simulink library "cpc5"  (R2016a)
settings: Solver=ode45  StartTime=0.0  StopTime=10.0  RelTol=1e-3
undefined symbols (not defined in the file): sMP
libraries: CPC5_SFUN_wrapper x1
settings Model: Creator=ploch37  LastModifiedBy=PLOCH37
settings DataIOCC: LimitDataPoints=on
settings DebuggingCC: AllowSymbolicDim=off

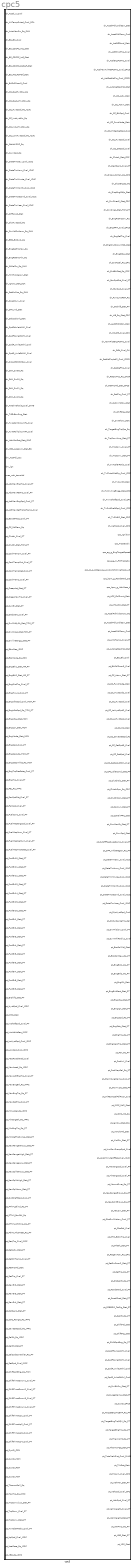
== system cpc5 ==
  cpc5 : Subsystem  mask{user_config=sMP.ctrl.cpc.user_config}
      mask prompts: user_config "Configuration String for S-Function"
      mask init:
      | cpc_mask_init;

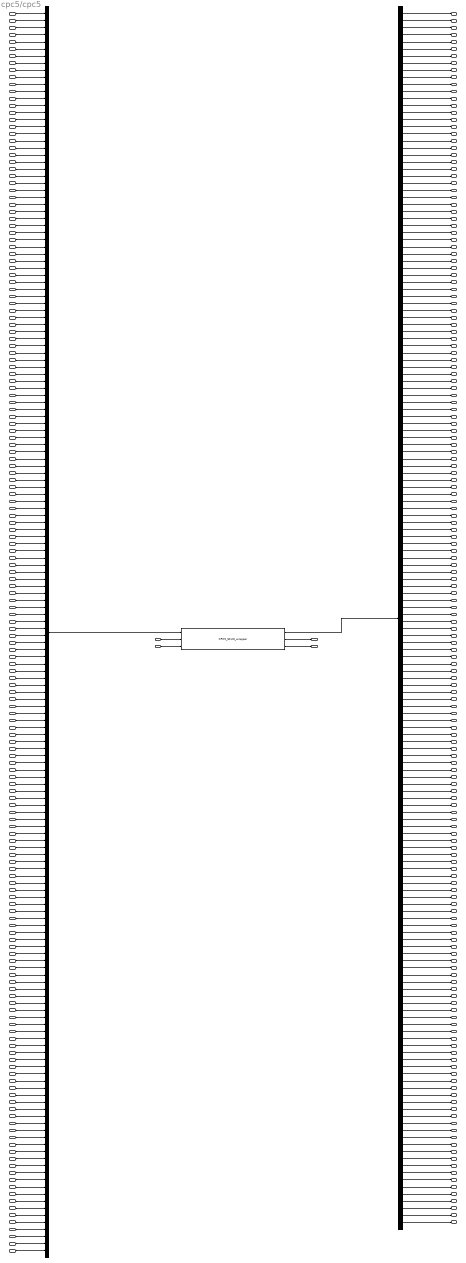
== system cpc5/cpc5 ==
  note: In- and Outports form a2lbus created with
      | cpc5_createPorts.m
      | from Spec folder in MKS.
      |
      | Ports sorted alphabetically with
      | slcSortPort.m
      | from tp/ead tools folder
  ch_Accel_X_Cval : Inport
  ch_AirTempOutsd_Cval_SCA : Inport  Port=2
  ch_AutoManSw_Rq_SAM : Inport  Port=3
  ch_BS_Brk_Cval : Inport  Port=4
  ch_BS_CSCPC_Acc_Stat : Inport  Port=5
  ch_BS_CSCPC_Intf_Stat : Inport  Port=6
  ch_BS_CSCPC_RqPerf_Stat : Inport  Port=7
  ch_BS_HB_RqPerf_Stat : Inport  Port=8
  ch_BrkPdlPosn3_Cval : Inport  Port=9
  ch_CC_DecHystSw_Rq : Inport  Port=10
  ch_CC_DecLoHystSw_Rq : Inport  Port=11
  ch_CC_HystSpd_Rq_ICUC : Inport  Port=12
  ch_CC_IncHystSw_Rq : Inport  Port=13
  ch_CC_IncLoHystSw_Rq : Inport  Port=14
  ch_CC_LowHystSpd_Rq_ICUC : Inport  Port=15
  ch_CstValIPPC_Rq : Inport  Port=16
  ch_CurvSpd_Rq : Inport  Port=17
  ch_DateTmDay_Cval_ICUC : Inport  Port=18
  ch_DateTmHour_Cval_ICUC : Inport  Port=19
  ch_DateTmMinute_Cval_ICUC : Inport  Port=20
  ch_DateTmMonth_Cval_ICUC : Inport  Port=21
  ch_DateTmSecond_Cval_ICUC : Inport  Port=22
  ch_DateTmYear_Cval_ICUC : Inport  Port=23
  ch_DiffLkIAC_Stat : Inport  Port=24
  ch_DipHystSpd_Rq : Inport  Port=25
  ch_DrvMdSwNorm_Rq_SAM : Inport  Port=26
  ch_EBS_BrkSw2_Rq : Inport  Port=27
  ch_EngRetTrqMax_Rq : Inport  Port=28
  ch_EngRetTrqMin_Rq : Inport  Port=29
  ch_GrSelSw_Rq_SAM : Inport  Port=30
  ch_HillHolderAvl_Stat : Inport  Port=31
  ch_IgnSw_Stat_SCA : Inport  Port=32
  ch_RetSwPos_Rq_SAM : Inport  Port=33
  ch_RoadCurv_Cval : Inport  Port=34
  ch_SFA_Ind_Stat : Inport  Port=35
  ch_SelSpdUnit_Stat : Inport  Port=36
  ch_SpdFtAxleLtWhl_Cval : Inport  Port=37
  ch_SpdFtAxleRtWhl_Cval : Inport  Port=38
  ch_SpdR_AxleLtWhl_Cval : Inport  Port=39
  ch_SpdR_AxleRtWhl_Cval : Inport  Port=40
  ch_SrcAdrBrkCtrlDev_Cval : Inport  Port=41
  ch_StW_Sw09_Rq : Inport  Port=42
  ch_StW_Sw10_Rq : Inport  Port=43
  ch_StW_Sw11_Rq : Inport  Port=44
  ch_StW_Sw13_Rq : Inport  Port=45
  ch_TotalVehDist_Cval_DIAG : Inport  Port=46
  ch_TrfGrBoxRng_Stat : Inport  Port=47
  ch_TyreRollCircumFA_Cval : Inport  Port=48
  ch_TyreRollCircumRA_Cval : Inport  Port=49
  ch_VehMtnDet_Stat_ICUC : Inport  Port=50
  ch_XBR_AccelLim_Stat_BS : Inport  Port=51
  drv_AccPdl_pos : Inport  Port=52
  drv_ign : Inport  Port=53
  mec_veh_transVel : Inport  Port=54
  pt_AbsMaxEngTrq_Cval_PT : Inport  Port=55
  pt_AbsMaxRetTrq_Cval_PT : Inport  Port=56
  pt_ActlMaxEngSpd_Cval_PT : Inport  Port=57
  pt_ActlMaxRetTrqNoTemp_Cval : Inport  Port=58
  pt_BoostPress_Cval_PT : Inport  Port=59
  pt_CC_MdDem_Rq : Inport  Port=60
  pt_Clutch_Cval_PT : Inport  Port=61
  pt_Clutch_Stat_TCM_PT : Inport  Port=62
  pt_CoolTempIn_Cval_PT : Inport  Port=63
  pt_CoolTempOut_Cval_PT : Inport  Port=64
  pt_CoolTempRet_Cval_PT : Inport  Port=65
  pt_CoolTemp_Cval_PT : Inport  Port=66
  pt_CreepAct_Stat_PT : Inport  Port=67
  pt_CreepMaxTrq_Cval_PT : Inport  Port=68
  pt_CurrGr_Stat_PT : Inport  Port=69
  pt_DeclSens_Cval_PT : Inport  Port=70
  pt_DrvDirByGr_Stat_TCM_PT : Inport  Port=71
  pt_DrvDirec_Stat_TCM_PT : Inport  Port=72
  pt_DrvlineEngg_Stat_PT : Inport  Port=73
  pt_EbmReq_IPPC : Inport  Port=74
  pt_EcoMode_Rq_PPC : Inport  Port=75
  pt_EngBrk1_Stat_MR_PT : Inport  Port=76
  pt_EngBrk2_Stat_MR_PT : Inport  Port=77
  pt_EngFrictTrq_Cval_PT : Inport  Port=78
  pt_EngHours_Cval_PT : Inport  Port=79
  pt_EngIdleSpd_Cval_MCM_PT : Inport  Port=80
  pt_EngIdleSpd_Rq_TCM_PT : Inport  Port=81
  pt_EngIdle_Stat_MCM : Inport  Port=82
  pt_EngIgn_Stat_MCM : Inport  Port=83
  pt_EngMode_Stat_MCM : Inport  Port=84
  pt_EngSpd_Cval_PT : Inport  Port=85
  pt_EngSpd_Rq_TCM_PT : Inport  Port=86
  pt_EngStSpInhbt_Rq_MCM : Inport  Port=87
  pt_EngTrqDecRate_Cval_PT : Inport  Port=88
  pt_EngTrq_Cval_PT : Inport  Port=89
  pt_FEL_Rq_IPPC : Inport  Port=90
  pt_FanSpdPct_Cval_PT : Inport  Port=91
  pt_FanSpd_Cval_PT : Inport  Port=92
  pt_FuelCons_Cval_PT : Inport  Port=93
  pt_FuelMapEngSpd_Cval_PT : Inport  Port=94
  pt_FuelMapNum_Cval_PT : Inport  Port=95
  pt_FuelMapSelNum_Cval_PT : Inport  Port=96
  pt_FuelMapTrqNoBst_Cval_PT : Inport  Port=97
  pt_FwdGr10_Stat_PT : Inport  Port=98
  pt_FwdGr11_Stat_PT : Inport  Port=99
  pt_FwdGr12_Stat_PT : Inport  Port=100
  pt_FwdGr13_Stat_PT : Inport  Port=101
  pt_FwdGr14_Stat_PT : Inport  Port=102
  pt_FwdGr15_Stat_PT : Inport  Port=103
  pt_FwdGr16_Stat_PT : Inport  Port=104
  pt_FwdGr1_Stat_PT : Inport  Port=105
  pt_FwdGr2_Stat_PT : Inport  Port=106
  pt_FwdGr3_Stat_PT : Inport  Port=107
  pt_FwdGr4_Stat_PT : Inport  Port=108
  pt_FwdGr5_Stat_PT : Inport  Port=109
  pt_FwdGr6_Stat_PT : Inport  Port=110
  pt_FwdGr7_Stat_PT : Inport  Port=111
  pt_FwdGr8_Stat_PT : Inport  Port=112
  pt_FwdGr9_Stat_PT : Inport  Port=113
  pt_GrShift_Stat_PT : Inport  Port=114
  pt_HystSpd_Cval_IPPC : Inport  Port=115
  pt_IPPC_Stat : Inport  Port=116
  pt_InShaftSpd_Cval_PT : Inport  Port=117
  pt_IntrUrbUcReq_IPPC : Inport  Port=118
  pt_LoHystSpd_Cval_IPPC : Inport  Port=119
  pt_LowSpd_Cval_IPPC : Inport  Port=120
  pt_MapRoadGrad_Cval : Inport  Port=121
  pt_MaxAccel_Rq_IPPC : Inport  Port=122
  pt_MaxActlEngTrq_Cval_PT : Inport  Port=123
  pt_MaxEngBrk_Rq_IPPC : Inport  Port=124
  pt_MaxEngTrq_Rq_PT : Inport  Port=125
  pt_MaxRetTrq_Cval_PT : Inport  Port=126
  pt_MinAccel_Rq_IPPC : Inport  Port=127
  pt_MinEngBrk_Rq_IPPC : Inport  Port=128
  pt_MinEngTrq_Rq_PT : Inport  Port=129
  pt_MinRetTrqPwrUp_Stat_PT : Inport  Port=130
  pt_NeuRangeGroup_Stat_PT : Inport  Port=131
  pt_NeuRangeHigh_Stat_PT : Inport  Port=132
  pt_NeuRangeLow_Stat_PT : Inport  Port=133
  pt_NeuSplitGroup_Stat_PT : Inport  Port=134
  pt_NeuSplitHigh_Stat_PT : Inport  Port=135
  pt_NeuSplitLow_Stat_PT : Inport  Port=136
  pt_OutShaftSpd_Cval_PT : Inport  Port=137
  pt_PThM_Blind_Rq_PT : Inport  Port=138
  pt_PThM_FanCtrl_Rq : Inport  Port=139
  pt_PThM_WtrPmp_Rq_PT : Inport  Port=140
  pt_PthM_ThstHeat_Rq_PT : Inport  Port=141
  pt_ReqTrq_Cval_IPPC : Inport  Port=142
  pt_RetActv_Stat_PT : Inport  Port=143
  pt_RetOilTemp_Cval_PT : Inport  Port=144
  pt_RetTrqMd_Stat : Inport  Port=145
  pt_RetTrq_Cval_PT : Inport  Port=146
  pt_RevGr2_Stat_PT : Inport  Port=147
  pt_RevGr3_Stat_PT : Inport  Port=148
  pt_RevGr4_Stat_PT : Inport  Port=149
  pt_RotSens_Stat_PT : Inport  Port=150
  pt_SOC_Range_Rq_IPPC : Inport  Port=151
  pt_SaveSetSpd_Rq_IPPC : Inport  Port=152
  pt_SelGr_Rq_IPPC : Inport  Port=153
  pt_SelGr_Stat_PT : Inport  Port=154
  pt_SelSpdController_Rq_PT : Inport  Port=155
  pt_SetSpd_Cval_IPPC : Inport  Port=156
  pt_ShiftSprtEng_Rq_TCM : Inport  Port=157
  pt_ShiftTimeDown1_Cval_PT : Inport  Port=158
  pt_ShiftTimeDown2_Cval_PT : Inport  Port=159
  pt_ShiftTimeDown3_Cval_PT : Inport  Port=160
  pt_ShiftTimeDown4_Cval_PT : Inport  Port=161
  pt_ShiftTimeUp1_Cval_PT : Inport  Port=162
  pt_ShiftTimeUp2_Cval_PT : Inport  Port=163
  pt_ShiftTimeUp3_Cval_PT : Inport  Port=164
  pt_ShiftTimeUp4_Cval_PT : Inport  Port=165
  pt_SysID_CCM : Inport  Port=166
  pt_SysID_MCM : Inport  Port=167
  pt_SysID_RCM : Inport  Port=168
  pt_SysID_TCM : Inport  Port=169
  pt_ThermoRoll_Rq : Inport  Port=170
  pt_TopTrq_Rq_IPPC : Inport  Port=171
  pt_TrqConvLkup_Stat_PT : Inport  Port=172
  pt_TrqConv_Cval_PT : Inport  Port=173
  pt_TrqConv_Stat_PT : Inport  Port=174
  pt_TxActlGrRatio_Cval_PT : Inport  Port=175
  pt_UpSpd_Cval_IPPC : Inport  Port=176
  pt_UseCase_Rq_IPPC : Inport  Port=177
  pt_XBR_Rq_IPPC : Inport  Port=178
  CPC5_SFUN_wrapper : CPC5_SFUN_wrapper/CPC5_SFUN_wrapper  SystemSampleTime=-1
  Inputs : BusCreator  Inputs=176
  Outputs : BusSelector  OutputSignals=out_ch_AccelPdlLoIdleSw_Stat,out_ch_AccelPdlPosn_Cval,out_ch_ActOffCond_Stat,out_ch_ActlEmotTrq_Cval,out_ch_ActlEngPctTrq_Cval,out_ch_ActlMaxAvlRetPctTrq_Cval_CPC3,out_ch_ActlRetPctTrq_Cval_CPC3,out_ch_AutoSetSpdMd_Stat,out_ch_CC_Actv_Stat,out_ch_CC_Actvn_Stat,out_ch_CC_BrkSpd_Cval,out_ch_CC_FuncMode_Stat,out_ch_CC_HiResSetSpd_Cval,out_ch_CC_HystSpd_Cval,out_ch_CC_SetSpd_Cval,out_ch_Clutch_Stat_CPC,out_ch_DeclSens_Cval_PT,out_ch_DispAutoMan_Rq_CPC,out_ch_DispEngSp_Rq,out_ch_DispEngStSp_Stat,out_ch_DrvDirec2_Stat_CPC,out_ch_DrvDirec_Stat_TCM_PT,out_ch_EngPctTrqDrv_Rq,out_ch_EngRPM_Cval_CPC3,out_ch_EngRefTrq_Cval,out_ch_EngShutDownMSS_Stat,out_ch_EngStSp_Stat,out_ch_ExtAccel_Rq_CPC,out_ch_ExtBrkStat_Rq_CPC,out_ch_FanSpdPct_Cval_PT,out_ch_FanSpd_Cval_PT,out_ch_FuncLmpRET_Rq,out_ch_GrShift_Stat_PT,out_ch_HB_Rq_Stat_CPC,out_ch_LastGrRlsRsn_Stat,out_ch_MC_E3_Cval_CPC,out_ch_NomFrictEngPctTrq_Cval,out_ch_PtRt_Cval_CH,out_ch_RetPctTrqActl2_Cval_CPC3,out_ch_RetRefTrq_Cval,out_ch_RetSwPos_Rq_STSR,out_ch_RetTrqMd_Stat_CPC3,out_ch_RetTrq_Cval_PT,out_ch_SLDrvMdSw_Stat,out_ch_ShiftPrg_Stat,out_ch_SrvBrkSw_Stat,out_ch_TargetEngTrqCpc_Rq,out_ch_TrqConvLkup_Stat_PT,out_ch_TrqConv_Cval_PT,out_ch_TrqConv_Stat_PT,out_ch_TxActlGrRatio_Cval,out_ch_TxClutchPctSlp_Cval_CPC,out_ch_TxCurrGr_Stat,out_ch_TxDrvlineEngg_Stat_CPC,out_ch_TxInShaftSpd_Cval_CPC,out_ch_TxOutShaftSpd_Cval_CPC,out_ch_TxShftIP_Stat_CPC,out_ch_VehSpd_Cval_CPC,out_pt_ACC_CtrlDmnt_Stat,out_pt_ATC_Ctrl_Stat_PT,out_pt_AccelPdlKickDnSw_Rq,out_pt_AccelPdlLoIdleSw_Stat,out_pt_AccelPdlPosn_Cval,out_pt_AmbTemp_Cval_PT,out_pt_AutoSetSpdMd_Stat,out_pt_BS_Brk_Cval,out_pt_BrkPdlPosn3_Cval,out_pt_CC_Actvn_Stat_PT,out_pt_CC_FuncMode_Stat,out_pt_CC_HystSpd2_Cval,out_pt_CC_HystSpd_Cval,out_pt_CC_LoHystSpd2_Cval,out_pt_CC_LoHystSpd_Cval,out_pt_CC_Md_Stat,out_pt_CC_SaveSetSpd_Rs,out_pt_CC_SetSpd3_Cval,out_pt_CC_SetSpd_Cval,out_pt_CC_SetSpd_Estm_Cval,out_pt_CPC_IdleCond_Stat_PT,out_pt_ClutchCls_Stat_PT,out_pt_ClutchOpn_Rq_CPC,out_pt_ClutchOpn_Stat_PT,out_pt_CoolLvl_Stat_PT,out_pt_CstValIPPC_Stat,out_pt_CurrManGr_Stat_PT,out_pt_CurvSpd_Stat,out_pt_CutoffFreqSurgDamp_Cval_PT,out_pt_DPF_InhbtRegen_Rq_PT,out_pt_DateTmDay_Cval_ICUC,out_pt_DateTmHour_Cval_ICUC,out_pt_DateTmMinute_Cval_ICUC,out_pt_DateTmMonth_Cval_ICUC,out_pt_DateTmSecond_Cval_ICUC,out_pt_DateTmYear_Cval_ICUC,out_pt_DipHystSpd_Cval,out_pt_DisturbanceTrq_Cal,out_pt_DrvFriction_Cval_PT,out_pt_DynWhlRadius_Cval,out_pt_EcoRollMd_Stat,out_pt_EcoRollNeu_Rq_PT,out_pt_EngBrk1_Rq_PT,out_pt_EngBrk2_Rq_PT,out_pt_EngCrk_Stat,out_pt_EngExtStart_Stat_PT,out_pt_EngIdle_Stat_PT,out_pt_EngIgn_Stat_PT,out_pt_EngSpd_Rq_PT,out_pt_EngStrtr_Stat_PT,out_pt_EngTrq_Rq_PT,out_pt_EngZeroTrq_Stat_PT,out_pt_Fan_Rq_PT,out_pt_FuelLvl_Cval,out_pt_FuelMapSel_Rq_PT,out_pt_GaimSurgDamp_Cval_PT,out_pt_GovType_Stat_PT,out_pt_HiResAccelPdlPosn_Cval,out_pt_IPPC_Md2_Stat,out_pt_IPPC_Md_Rq,out_pt_IgnSw_Stat_SCA,out_pt_IntrUrbMd_Stat,out_pt_KickDn_Stat_PT,out_pt_LimGovDroopSpd_Cval,out_pt_LocalMinuteOffset_Cval_ICUC,out_pt_MaxEngSpd_Cval_PT,out_pt_MinEngSpd_Cval_PT,out_pt_MomntOver_Rq_PT,out_pt_NeuRangeGroup_Rq_PT,out_pt_NeuSplitGroup_Rq_PT,out_pt_NeuSw_Stat_PT,out_pt_ObsDrvFriction_Cval_PT,out_pt_ObsSel_Cval,out_pt_PTO_EstmTrq_Cval,out_pt_PrkBrk_Stat_PT,out_pt_RegenActv_Rq_CPC,out_pt_RetSwPosn2_Stat_PT,out_pt_RetTrq_Rq_PT,out_pt_RlsSelGr_Rq_PT,out_pt_RoadGrad_Cval_PT,out_pt_RoadGrad_Stat_PT,out_pt_SPEEDO_ZeSig_Stat_PT,out_pt_SelGr_Rq_PT,out_pt_ShiftMd_Stat,out_pt_ShiftPrg_Stat,out_pt_ShiftSprtEng_Rq_PT,out_pt_SpdFtAxleLtWhl_Cval,out_pt_SpdFtAxleRtWhl_Cval,out_pt_SpdR_AxleLtWhl_Cval,out_pt_SpdR_AxleRtWhl_Cval,out_pt_SrvBrkSw_Stat_PT,out_pt_SurgeDamp_Stat_PT,out_pt_SysID_CPC3,out_pt_TargetEngTrqETP_Rq_PT,out_pt_TargetEngTrqRQV_Rq_PT,out_pt_TargetEngTrq_Rq_PT,out_pt_ThermoHt_Rq_PT,out_pt_ThermoMgt_Stat_PT,out_pt_TotalVehDist_Cval_DIAG,out_pt_TrlrDet_Stat,out_pt_TrqLim_Cval_CPC,out_pt_VehMtn_Stat_PT,out_pt_VehSpd_Cval_CPC,out_pt_VehSpd_Cval_PT,out_pt_VehWeight_Cval_PT,out_pt_VehWeight_Stat_PT,out_pt_WtrPmp_Rq_PT,out_pt_XBR_Stat_PT,out_pt_XSS_Stat,out_cpc_Ignition,out_cpc_TrqDecIdx,out_cpc_ag_g_EngTargetSpeed,out_cpc_ag_m_FiltTrqRatio,out_cpc_cc_p_CcSecure_LowSwitchOnVehSpd_u8
  ch_AccelPdlLoIdleSw_Stat : Outport
  ch_AccelPdlPosn_Cval : Outport  Port=2
  ch_ActOffCond_Stat : Outport  Port=3
  ch_ActlEmotTrq_Cval : Outport  Port=4
  ch_ActlEngPctTrq_Cval : Outport  Port=5
  ch_ActlMaxAvlRetPctTrq_Cval_CPC3 : Outport  Port=6
  ch_ActlRetPctTrq_Cval_CPC3 : Outport  Port=7
  ch_AutoSetSpdMd_Stat : Outport  Port=8
  ch_CC_Actv_Stat : Outport  Port=9
  ch_CC_Actvn_Stat : Outport  Port=10
  ch_CC_BrkSpd_Cval : Outport  Port=11
  ch_CC_FuncMode_Stat : Outport  Port=12
  ch_CC_HiResSetSpd_Cval : Outport  Port=13
  ch_CC_HystSpd_Cval : Outport  Port=14
  ch_CC_SetSpd_Cval : Outport  Port=15
  ch_Clutch_Stat_CPC : Outport  Port=16
  ch_DeclSens_Cval_PT : Outport  Port=17
  ch_DispAutoMan_Rq_CPC : Outport  Port=18
  ch_DispEngSp_Rq : Outport  Port=19
  ch_DispEngStSp_Stat : Outport  Port=20
  ch_DrvDirec2_Stat_CPC : Outport  Port=21
  ch_DrvDirec_Stat_TCM_PT : Outport  Port=22
  ch_EngPctTrqDrv_Rq : Outport  Port=23
  ch_EngRPM_Cval_CPC3 : Outport  Port=24
  ch_EngRefTrq_Cval : Outport  Port=25
  ch_EngShutDownMSS_Stat : Outport  Port=26
  ch_EngStSp_Stat : Outport  Port=27
  ch_ExtAccel_Rq_CPC : Outport  Port=28
  ch_ExtBrkStat_Rq_CPC : Outport  Port=29
  ch_FanSpdPct_Cval_PT : Outport  Port=30
  ch_FanSpd_Cval_PT : Outport  Port=31
  ch_FuncLmpRET_Rq : Outport  Port=32
  ch_GrShift_Stat_PT : Outport  Port=33
  ch_HB_Rq_Stat_CPC : Outport  Port=34
  ch_LastGrRlsRsn_Stat : Outport  Port=35
  ch_MC_E3_Cval_CPC : Outport  Port=36
  ch_NomFrictEngPctTrq_Cval : Outport  Port=37
  ch_PtRt_Cval_CH : Outport  Port=38
  ch_RetPctTrqActl2_Cval_CPC3 : Outport  Port=39
  ch_RetRefTrq_Cval : Outport  Port=40
  ch_RetSwPos_Rq_STSR : Outport  Port=41
  ch_RetTrqMd_Stat_CPC3 : Outport  Port=42
  ch_RetTrq_Cval_PT : Outport  Port=43
  ch_SLDrvMdSw_Stat : Outport  Port=44
  ch_ShiftPrg_Stat : Outport  Port=45
  ch_SrvBrkSw_Stat : Outport  Port=46
  ch_TargetEngTrqCpc_Rq : Outport  Port=47
  ch_TrqConvLkup_Stat_PT : Outport  Port=48
  ch_TrqConv_Cval_PT : Outport  Port=49
  ch_TrqConv_Stat_PT : Outport  Port=50
  ch_TxActlGrRatio_Cval : Outport  Port=51
  ch_TxClutchPctSlp_Cval_CPC : Outport  Port=52
  ch_TxCurrGr_Stat : Outport  Port=53
  ch_TxDrvlineEngg_Stat_CPC : Outport  Port=54
  ch_TxInShaftSpd_Cval_CPC : Outport  Port=55
  ch_TxOutShaftSpd_Cval_CPC : Outport  Port=56
  ch_TxShftIP_Stat_CPC : Outport  Port=57
  ch_VehSpd_Cval_CPC : Outport  Port=58
  cpc_Ignition : Outport  Port=59
  cpc_TrqDecIdx : Outport  Port=60
  cpc_ag_g_EngTargetSpeed : Outport  Port=61
  cpc_ag_m_FiltTrqRatio : Outport  Port=62
  cpc_cc_p_CcSecure_LowSwitchOnVehSpd_u8 : Outport  Port=63
  cpc_itpm_g_RoadGrad_pct : Outport  Port=64
  cpc_itpm_g_VehMass_t : Outport  Port=65
  pt_ACC_CtrlDmnt_Stat : Outport  Port=66
  pt_ATC_Ctrl_Stat_PT : Outport  Port=67
  pt_AccelPdlKickDnSw_Rq : Outport  Port=68
  pt_AccelPdlLoIdleSw_Stat : Outport  Port=69
  pt_AccelPdlPosn_Cval : Outport  Port=70
  pt_AmbTemp_Cval_PT : Outport  Port=71
  pt_AutoSetSpdMd_Stat : Outport  Port=72
  pt_BS_Brk_Cval : Outport  Port=73
  pt_BrkPdlPosn3_Cval : Outport  Port=74
  pt_CC_Actvn_Stat_PT : Outport  Port=75
  pt_CC_FuncMode_Stat : Outport  Port=76
  pt_CC_HystSpd2_Cval : Outport  Port=77
  pt_CC_HystSpd_Cval : Outport  Port=78
  pt_CC_LoHystSpd2_Cval : Outport  Port=79
  pt_CC_LoHystSpd_Cval : Outport  Port=80
  pt_CC_Md_Stat : Outport  Port=81
  pt_CC_SaveSetSpd_Rs : Outport  Port=82
  pt_CC_SetSpd3_Cval : Outport  Port=83
  pt_CC_SetSpd_Cval : Outport  Port=84
  pt_CC_SetSpd_Estm_Cval : Outport  Port=85
  pt_CPC_IdleCond_Stat_PT : Outport  Port=86
  pt_ClutchCls_Stat_PT : Outport  Port=87
  pt_ClutchOpn_Rq_CPC : Outport  Port=88
  pt_ClutchOpn_Stat_PT : Outport  Port=89
  pt_CoolLvl_Stat_PT : Outport  Port=90
  pt_CstValIPPC_Stat : Outport  Port=91
  pt_CurrManGr_Stat_PT : Outport  Port=92
  pt_CurvSpd_Stat : Outport  Port=93
  pt_CutoffFreqSurgDamp_Cval_PT : Outport  Port=94
  pt_DPF_InhbtRegen_Rq_PT : Outport  Port=95
  pt_DateTmDay_Cval_ICUC : Outport  Port=96
  pt_DateTmHour_Cval_ICUC : Outport  Port=97
  pt_DateTmMinute_Cval_ICUC : Outport  Port=98
  pt_DateTmMonth_Cval_ICUC : Outport  Port=99
  pt_DateTmSecond_Cval_ICUC : Outport  Port=100
  pt_DateTmYear_Cval_ICUC : Outport  Port=101
  pt_DipHystSpd_Cval : Outport  Port=102
  pt_DisturbanceTrq_Cal : Outport  Port=103
  pt_DrvFriction_Cval_PT : Outport  Port=104
  pt_DynWhlRadius_Cval : Outport  Port=105
  pt_EcoRollMd_Stat : Outport  Port=106
  pt_EcoRollNeu_Rq_PT : Outport  Port=107
  pt_EngBrk1_Rq_PT : Outport  Port=108
  pt_EngBrk2_Rq_PT : Outport  Port=109
  pt_EngCrk_Stat : Outport  Port=110
  pt_EngExtStart_Stat_PT : Outport  Port=111
  pt_EngIdle_Stat_PT : Outport  Port=112
  pt_EngIgn_Stat_PT : Outport  Port=113
  pt_EngSpd_Rq_PT : Outport  Port=114
  pt_EngStrtr_Stat_PT : Outport  Port=115
  pt_EngTrq_Rq_PT : Outport  Port=116
  pt_EngZeroTrq_Stat_PT : Outport  Port=117
  pt_Fan_Rq_PT : Outport  Port=118
  pt_FuelLvl_Cval : Outport  Port=119
  pt_FuelMapSel_Rq_PT : Outport  Port=120
  pt_GaimSurgDamp_Cval_PT : Outport  Port=121
  pt_GovType_Stat_PT : Outport  Port=122
  pt_HiResAccelPdlPosn_Cval : Outport  Port=123
  pt_IPPC_Md2_Stat : Outport  Port=124
  pt_IPPC_Md_Rq : Outport  Port=125
  pt_IgnSw_Stat_SCA : Outport  Port=126
  pt_IntrUrbMd_Stat : Outport  Port=127
  pt_KickDn_Stat_PT : Outport  Port=128
  pt_LimGovDroopSpd_Cval : Outport  Port=129
  pt_LocalMinuteOffset_Cval_ICUC : Outport  Port=130
  pt_MaxEngSpd_Cval_PT : Outport  Port=131
  pt_MinEngSpd_Cval_PT : Outport  Port=132
  pt_MomntOver_Rq_PT : Outport  Port=133
  pt_NeuRangeGroup_Rq_PT : Outport  Port=134
  pt_NeuSplitGroup_Rq_PT : Outport  Port=135
  pt_NeuSw_Stat_PT : Outport  Port=136
  pt_ObsDrvFriction_Cval_PT : Outport  Port=137
  pt_ObsSel_Cval : Outport  Port=138
  pt_PTO_EstmTrq_Cval : Outport  Port=139
  pt_PrkBrk_Stat_PT : Outport  Port=140
  pt_RegenActv_Rq_CPC : Outport  Port=141
  pt_RetSwPosn2_Stat_PT : Outport  Port=142
  pt_RetTrq_Rq_PT : Outport  Port=143
  pt_RlsSelGr_Rq_PT : Outport  Port=144
  pt_RoadGrad_Cval_PT : Outport  Port=145
  pt_RoadGrad_Stat_PT : Outport  Port=146
  pt_SPEEDO_ZeSig_Stat_PT : Outport  Port=147
  pt_SelGr_Rq_PT : Outport  Port=148
  pt_ShiftMd_Stat : Outport  Port=149
  pt_ShiftPrg_Stat : Outport  Port=150
  pt_ShiftSprtEng_Rq_PT : Outport  Port=151
  pt_SpdFtAxleLtWhl_Cval : Outport  Port=152
  pt_SpdFtAxleRtWhl_Cval : Outport  Port=153
  pt_SpdR_AxleLtWhl_Cval : Outport  Port=154
  pt_SpdR_AxleRtWhl_Cval : Outport  Port=155
  pt_SrvBrkSw_Stat_PT : Outport  Port=156
  pt_SurgeDamp_Stat_PT : Outport  Port=157
  pt_SysID_CPC3 : Outport  Port=158
  pt_TargetEngTrqETP_Rq_PT : Outport  Port=159
  pt_TargetEngTrqRQV_Rq_PT : Outport  Port=160
  pt_TargetEngTrq_Rq_PT : Outport  Port=161
  pt_ThermoHt_Rq_PT : Outport  Port=162
  pt_ThermoMgt_Stat_PT : Outport  Port=163
  pt_TotalVehDist_Cval_DIAG : Outport  Port=164
  pt_TrlrDet_Stat : Outport  Port=165
  pt_TrqLim_Cval_CPC : Outport  Port=166
  pt_VehMtn_Stat_PT : Outport  Port=167
  pt_VehSpd_Cval_CPC : Outport  Port=168
  pt_VehSpd_Cval_PT : Outport  Port=169
  pt_VehWeight_Cval_PT : Outport  Port=170
  pt_VehWeight_Stat_PT : Outport  Port=171
  pt_WtrPmp_Rq_PT : Outport  Port=172
  pt_XBR_Stat_PT : Outport  Port=173
  pt_XSS_Stat : Outport  Port=174
  wires:
  drv_AccPdl_pos/1 -> CPC5_SFUN_wrapper/2
  mec_veh_transVel/1 -> CPC5_SFUN_wrapper/3
  CPC5_SFUN_wrapper/2 -> cpc_itpm_g_RoadGrad_pct/1
  CPC5_SFUN_wrapper/3 -> cpc_itpm_g_VehMass_t/1
  ch_Accel_X_Cval/1 -> Inputs/1  "ch_Accel_X_Cval"
  ch_AirTempOutsd_Cval_SCA/1 -> Inputs/2  "ch_AirTempOutsd_Cval_SCA"
  ch_AutoManSw_Rq_SAM/1 -> Inputs/3  "ch_AutoManSw_Rq_SAM"
  ch_BS_Brk_Cval/1 -> Inputs/4  "ch_BS_Brk_Cval"
  ch_BS_CSCPC_Acc_Stat/1 -> Inputs/5  "ch_BS_CSCPC_Acc_Stat"
  ch_BS_CSCPC_Intf_Stat/1 -> Inputs/6  "ch_BS_CSCPC_Intf_Stat"
  ch_BS_CSCPC_RqPerf_Stat/1 -> Inputs/7  "ch_BS_CSCPC_RqPerf_Stat"
  ch_BS_HB_RqPerf_Stat/1 -> Inputs/8  "ch_BS_HB_RqPerf_Stat"
  ch_BrkPdlPosn3_Cval/1 -> Inputs/9  "ch_BrkPdlPosn3_Cval"
  ch_CC_DecHystSw_Rq/1 -> Inputs/10  "ch_CC_DecHystSw_Rq"
  ch_CC_DecLoHystSw_Rq/1 -> Inputs/11  "ch_CC_DecLoHystSw_Rq"
  ch_CC_HystSpd_Rq_ICUC/1 -> Inputs/12  "ch_CC_HystSpd_Rq_ICUC"
  ch_CC_IncHystSw_Rq/1 -> Inputs/13  "ch_CC_IncHystSw_Rq"
  ch_CC_IncLoHystSw_Rq/1 -> Inputs/14  "ch_CC_IncLoHystSw_Rq"
  ch_CC_LowHystSpd_Rq_ICUC/1 -> Inputs/15  "ch_CC_LowHystSpd_Rq_ICUC"
  ch_CstValIPPC_Rq/1 -> Inputs/16  "ch_CstValIPPC_Rq"
  ch_CurvSpd_Rq/1 -> Inputs/17  "ch_CurvSpd_Rq"
  ch_DateTmDay_Cval_ICUC/1 -> Inputs/18  "ch_DateTmDay_Cval_ICUC"
  ch_DateTmHour_Cval_ICUC/1 -> Inputs/19  "ch_DateTmHour_Cval_ICUC"
  ch_DateTmMinute_Cval_ICUC/1 -> Inputs/20  "ch_DateTmMinute_Cval_ICUC"
  ch_DateTmMonth_Cval_ICUC/1 -> Inputs/21  "ch_DateTmMonth_Cval_ICUC"
  ch_DateTmSecond_Cval_ICUC/1 -> Inputs/22  "ch_DateTmSecond_Cval_ICUC"
  ch_DateTmYear_Cval_ICUC/1 -> Inputs/23  "ch_DateTmYear_Cval_ICUC"
  ch_DiffLkIAC_Stat/1 -> Inputs/24  "ch_DiffLkIAC_Stat"
  ch_DipHystSpd_Rq/1 -> Inputs/25  "ch_DipHystSpd_Rq"
  ch_DrvMdSwNorm_Rq_SAM/1 -> Inputs/26  "ch_DrvMdSwNorm_Rq_SAM"
  ch_EBS_BrkSw2_Rq/1 -> Inputs/27  "ch_EBS_BrkSw2_Rq"
  ch_EngRetTrqMax_Rq/1 -> Inputs/28  "ch_EngRetTrqMax_Rq"
  ch_EngRetTrqMin_Rq/1 -> Inputs/29  "ch_EngRetTrqMin_Rq"
  ch_GrSelSw_Rq_SAM/1 -> Inputs/30  "ch_GrSelSw_Rq_SAM"
  ch_HillHolderAvl_Stat/1 -> Inputs/31  "ch_HillHolderAvl_Stat"
  ch_IgnSw_Stat_SCA/1 -> Inputs/32  "ch_IgnSw_Stat_SCA"
  ch_RetSwPos_Rq_SAM/1 -> Inputs/33  "ch_RetSwPos_Rq_SAM"
  ch_RoadCurv_Cval/1 -> Inputs/34  "ch_RoadCurv_Cval"
  ch_SFA_Ind_Stat/1 -> Inputs/35  "ch_SFA_Ind_Stat"
  ch_SelSpdUnit_Stat/1 -> Inputs/36  "ch_SelSpdUnit_Stat"
  ch_SpdFtAxleLtWhl_Cval/1 -> Inputs/37  "ch_SpdFtAxleLtWhl_Cval"
  ch_SpdFtAxleRtWhl_Cval/1 -> Inputs/38  "ch_SpdFtAxleRtWhl_Cval"
  ch_SpdR_AxleLtWhl_Cval/1 -> Inputs/39  "ch_SpdR_AxleLtWhl_Cval"
  ch_SpdR_AxleRtWhl_Cval/1 -> Inputs/40  "ch_SpdR_AxleRtWhl_Cval"
  ch_SrcAdrBrkCtrlDev_Cval/1 -> Inputs/41  "ch_SrcAdrBrkCtrlDev_Cval"
  ch_StW_Sw09_Rq/1 -> Inputs/42  "ch_StW_Sw09_Rq"
  ch_StW_Sw10_Rq/1 -> Inputs/43  "ch_StW_Sw10_Rq"
  ch_StW_Sw11_Rq/1 -> Inputs/44  "ch_StW_Sw11_Rq"
  ch_StW_Sw13_Rq/1 -> Inputs/45  "ch_StW_Sw13_Rq"
  ch_TotalVehDist_Cval_DIAG/1 -> Inputs/46  "ch_TotalVehDist_Cval_DIAG"
  ch_TrfGrBoxRng_Stat/1 -> Inputs/47  "ch_TrfGrBoxRng_Stat"
  ch_TyreRollCircumFA_Cval/1 -> Inputs/48  "ch_TyreRollCircumFA_Cval"
  ch_TyreRollCircumRA_Cval/1 -> Inputs/49  "ch_TyreRollCircumRA_Cval"
  ch_VehMtnDet_Stat_ICUC/1 -> Inputs/50  "ch_VehMtnDet_Stat_ICUC"
  ch_XBR_AccelLim_Stat_BS/1 -> Inputs/51  "ch_XBR_AccelLim_Stat_BS"
  pt_AbsMaxEngTrq_Cval_PT/1 -> Inputs/52  "pt_AbsMaxEngTrq_Cval_PT"
  pt_AbsMaxRetTrq_Cval_PT/1 -> Inputs/53  "pt_AbsMaxRetTrq_Cval_PT"
  pt_ActlMaxEngSpd_Cval_PT/1 -> Inputs/54  "pt_ActlMaxEngSpd_Cval_PT"
  pt_ActlMaxRetTrqNoTemp_Cval/1 -> Inputs/55  "pt_ActlMaxRetTrqNoTemp_Cval"
  pt_BoostPress_Cval_PT/1 -> Inputs/56  "pt_BoostPress_Cval_PT"
  pt_CC_MdDem_Rq/1 -> Inputs/57  "pt_CC_MdDem_Rq"
  pt_Clutch_Cval_PT/1 -> Inputs/58  "pt_Clutch_Cval_PT"
  pt_Clutch_Stat_TCM_PT/1 -> Inputs/59  "pt_Clutch_Stat_TCM_PT"
  pt_CoolTempIn_Cval_PT/1 -> Inputs/60  "pt_CoolTempIn_Cval_PT"
  pt_CoolTempOut_Cval_PT/1 -> Inputs/61  "pt_CoolTempOut_Cval_PT"
  pt_CoolTempRet_Cval_PT/1 -> Inputs/62  "pt_CoolTempRet_Cval_PT"
  pt_CoolTemp_Cval_PT/1 -> Inputs/63  "pt_CoolTemp_Cval_PT"
  pt_CreepAct_Stat_PT/1 -> Inputs/64  "pt_CreepAct_Stat_PT"
  pt_CreepMaxTrq_Cval_PT/1 -> Inputs/65  "pt_CreepMaxTrq_Cval_PT"
  pt_CurrGr_Stat_PT/1 -> Inputs/66  "pt_CurrGr_Stat_PT"
  pt_DeclSens_Cval_PT/1 -> Inputs/67  "pt_DeclSens_Cval_PT"
  pt_DrvDirByGr_Stat_TCM_PT/1 -> Inputs/68  "pt_DrvDirByGr_Stat_TCM_PT"
  pt_DrvDirec_Stat_TCM_PT/1 -> Inputs/69  "pt_DrvDirec_Stat_TCM_PT"
  pt_DrvlineEngg_Stat_PT/1 -> Inputs/70  "pt_DrvlineEngg_Stat_PT"
  pt_EbmReq_IPPC/1 -> Inputs/71  "pt_EbmReq_IPPC"
  pt_EcoMode_Rq_PPC/1 -> Inputs/72  "pt_EcoMode_Rq_PPC"
  pt_EngBrk1_Stat_MR_PT/1 -> Inputs/73  "pt_EngBrk1_Stat_MR_PT"
  pt_EngBrk2_Stat_MR_PT/1 -> Inputs/74  "pt_EngBrk2_Stat_MR_PT"
  pt_EngFrictTrq_Cval_PT/1 -> Inputs/75  "pt_EngFrictTrq_Cval_PT"
  pt_EngHours_Cval_PT/1 -> Inputs/76  "pt_EngHours_Cval_PT"
  pt_EngIdleSpd_Cval_MCM_PT/1 -> Inputs/77  "pt_EngIdleSpd_Cval_MCM_PT"
  pt_EngIdleSpd_Rq_TCM_PT/1 -> Inputs/78  "pt_EngIdleSpd_Rq_TCM_PT"
  pt_EngIdle_Stat_MCM/1 -> Inputs/79  "pt_EngIdle_Stat_MCM"
  pt_EngIgn_Stat_MCM/1 -> Inputs/80  "pt_EngIgn_Stat_MCM"
  pt_EngMode_Stat_MCM/1 -> Inputs/81  "pt_EngMode_Stat_MCM"
  pt_EngSpd_Cval_PT/1 -> Inputs/82  "pt_EngSpd_Cval_PT"
  pt_EngSpd_Rq_TCM_PT/1 -> Inputs/83  "pt_EngSpd_Rq_TCM_PT"
  pt_EngStSpInhbt_Rq_MCM/1 -> Inputs/84  "pt_EngStSpInhbt_Rq_MCM"
  pt_EngTrqDecRate_Cval_PT/1 -> Inputs/85  "pt_EngTrqDecRate_Cval_PT"
  pt_EngTrq_Cval_PT/1 -> Inputs/86  "pt_EngTrq_Cval_PT"
  pt_FEL_Rq_IPPC/1 -> Inputs/87  "pt_FEL_Rq_IPPC"
  pt_FanSpdPct_Cval_PT/1 -> Inputs/88  "pt_FanSpdPct_Cval_PT"
  pt_FanSpd_Cval_PT/1 -> Inputs/89  "pt_FanSpd_Cval_PT"
  pt_FuelCons_Cval_PT/1 -> Inputs/90  "pt_FuelCons_Cval_PT"
  pt_FuelMapEngSpd_Cval_PT/1 -> Inputs/91  "pt_FuelMapEngSpd_Cval_PT"
  pt_FuelMapNum_Cval_PT/1 -> Inputs/92  "pt_FuelMapNum_Cval_PT"
  pt_FuelMapSelNum_Cval_PT/1 -> Inputs/93  "pt_FuelMapSelNum_Cval_PT"
  pt_FuelMapTrqNoBst_Cval_PT/1 -> Inputs/94  "pt_FuelMapTrqNoBst_Cval_PT"
  pt_FwdGr10_Stat_PT/1 -> Inputs/95  "pt_FwdGr10_Stat_PT"
  pt_FwdGr11_Stat_PT/1 -> Inputs/96  "pt_FwdGr11_Stat_PT"
  pt_FwdGr12_Stat_PT/1 -> Inputs/97  "pt_FwdGr12_Stat_PT"
  pt_FwdGr13_Stat_PT/1 -> Inputs/98  "pt_FwdGr13_Stat_PT"
  pt_FwdGr14_Stat_PT/1 -> Inputs/99  "pt_FwdGr14_Stat_PT"
  pt_FwdGr15_Stat_PT/1 -> Inputs/100  "pt_FwdGr15_Stat_PT"
  pt_FwdGr16_Stat_PT/1 -> Inputs/101  "pt_FwdGr16_Stat_PT"
  pt_FwdGr1_Stat_PT/1 -> Inputs/102  "pt_FwdGr1_Stat_PT"
  pt_FwdGr2_Stat_PT/1 -> Inputs/103  "pt_FwdGr2_Stat_PT"
  pt_FwdGr3_Stat_PT/1 -> Inputs/104  "pt_FwdGr3_Stat_PT"
  pt_FwdGr4_Stat_PT/1 -> Inputs/105  "pt_FwdGr4_Stat_PT"
  pt_FwdGr5_Stat_PT/1 -> Inputs/106  "pt_FwdGr5_Stat_PT"
  pt_FwdGr6_Stat_PT/1 -> Inputs/107  "pt_FwdGr6_Stat_PT"
  pt_FwdGr7_Stat_PT/1 -> Inputs/108  "pt_FwdGr7_Stat_PT"
  pt_FwdGr8_Stat_PT/1 -> Inputs/109  "pt_FwdGr8_Stat_PT"
  pt_FwdGr9_Stat_PT/1 -> Inputs/110  "pt_FwdGr9_Stat_PT"
  pt_GrShift_Stat_PT/1 -> Inputs/111  "pt_GrShift_Stat_PT"
  pt_HystSpd_Cval_IPPC/1 -> Inputs/112  "pt_HystSpd_Cval_IPPC"
  pt_IPPC_Stat/1 -> Inputs/113  "pt_IPPC_Stat"
  pt_InShaftSpd_Cval_PT/1 -> Inputs/114  "pt_InShaftSpd_Cval_PT"
  pt_IntrUrbUcReq_IPPC/1 -> Inputs/115  "pt_IntrUrbUcReq_IPPC"
  pt_LoHystSpd_Cval_IPPC/1 -> Inputs/116  "pt_LoHystSpd_Cval_IPPC"
  pt_LowSpd_Cval_IPPC/1 -> Inputs/117  "pt_LowSpd_Cval_IPPC"
  pt_MapRoadGrad_Cval/1 -> Inputs/118  "pt_MapRoadGrad_Cval"
  pt_MaxAccel_Rq_IPPC/1 -> Inputs/119  "pt_MaxAccel_Rq_IPPC"
  pt_MaxActlEngTrq_Cval_PT/1 -> Inputs/120  "pt_MaxActlEngTrq_Cval_PT"
  pt_MaxEngBrk_Rq_IPPC/1 -> Inputs/121  "pt_MaxEngBrk_Rq_IPPC"
  pt_MaxEngTrq_Rq_PT/1 -> Inputs/122  "pt_MaxEngTrq_Rq_PT"
  pt_MaxRetTrq_Cval_PT/1 -> Inputs/123  "pt_MaxRetTrq_Cval_PT"
  pt_MinAccel_Rq_IPPC/1 -> Inputs/124  "pt_MinAccel_Rq_IPPC"
  pt_MinEngBrk_Rq_IPPC/1 -> Inputs/125  "pt_MinEngBrk_Rq_IPPC"
  pt_MinEngTrq_Rq_PT/1 -> Inputs/126  "pt_MinEngTrq_Rq_PT"
  pt_MinRetTrqPwrUp_Stat_PT/1 -> Inputs/127  "pt_MinRetTrqPwrUp_Stat_PT"
  pt_NeuRangeGroup_Stat_PT/1 -> Inputs/128  "pt_NeuRangeGroup_Stat_PT"
  pt_NeuRangeHigh_Stat_PT/1 -> Inputs/129  "pt_NeuRangeHigh_Stat_PT"
  pt_NeuRangeLow_Stat_PT/1 -> Inputs/130  "pt_NeuRangeLow_Stat_PT"
  pt_NeuSplitGroup_Stat_PT/1 -> Inputs/131  "pt_NeuSplitGroup_Stat_PT"
  pt_NeuSplitHigh_Stat_PT/1 -> Inputs/132  "pt_NeuSplitHigh_Stat_PT"
  pt_NeuSplitLow_Stat_PT/1 -> Inputs/133  "pt_NeuSplitLow_Stat_PT"
  pt_OutShaftSpd_Cval_PT/1 -> Inputs/134  "pt_OutShaftSpd_Cval_PT"
  pt_PThM_Blind_Rq_PT/1 -> Inputs/135  "pt_PThM_Blind_Rq_PT"
  pt_PThM_FanCtrl_Rq/1 -> Inputs/136  "pt_PThM_FanCtrl_Rq"
  pt_PThM_WtrPmp_Rq_PT/1 -> Inputs/137  "pt_PThM_WtrPmp_Rq_PT"
  pt_PthM_ThstHeat_Rq_PT/1 -> Inputs/138  "pt_PthM_ThstHeat_Rq_PT"
  pt_ReqTrq_Cval_IPPC/1 -> Inputs/139  "pt_ReqTrq_Cval_IPPC"
  pt_RetActv_Stat_PT/1 -> Inputs/140  "pt_RetActv_Stat_PT"
  pt_RetOilTemp_Cval_PT/1 -> Inputs/141  "pt_RetOilTemp_Cval_PT"
  pt_RetTrqMd_Stat/1 -> Inputs/142  "pt_RetTrqMd_Stat"
  pt_RetTrq_Cval_PT/1 -> Inputs/143  "pt_RetTrq_Cval_PT"
  pt_RevGr2_Stat_PT/1 -> Inputs/144  "pt_RevGr2_Stat_PT"
  pt_RevGr3_Stat_PT/1 -> Inputs/145  "pt_RevGr3_Stat_PT"
  pt_RevGr4_Stat_PT/1 -> Inputs/146  "pt_RevGr4_Stat_PT"
  pt_RotSens_Stat_PT/1 -> Inputs/147  "pt_RotSens_Stat_PT"
  pt_SOC_Range_Rq_IPPC/1 -> Inputs/148  "pt_SOC_Range_Rq_IPPC"
  pt_SaveSetSpd_Rq_IPPC/1 -> Inputs/149  "pt_SaveSetSpd_Rq_IPPC"
  pt_SelGr_Rq_IPPC/1 -> Inputs/150  "pt_SelGr_Rq_IPPC"
  pt_SelGr_Stat_PT/1 -> Inputs/151  "pt_SelGr_Stat_PT"
  pt_SelSpdController_Rq_PT/1 -> Inputs/152  "pt_SelSpdController_Rq_PT"
  pt_SetSpd_Cval_IPPC/1 -> Inputs/153  "pt_SetSpd_Cval_IPPC"
  pt_ShiftSprtEng_Rq_TCM/1 -> Inputs/154  "pt_ShiftSprtEng_Rq_TCM"
  pt_ShiftTimeDown1_Cval_PT/1 -> Inputs/155  "pt_ShiftTimeDown1_Cval_PT"
  pt_ShiftTimeDown2_Cval_PT/1 -> Inputs/156  "pt_ShiftTimeDown2_Cval_PT"
  pt_ShiftTimeDown3_Cval_PT/1 -> Inputs/157  "pt_ShiftTimeDown3_Cval_PT"
  pt_ShiftTimeDown4_Cval_PT/1 -> Inputs/158  "pt_ShiftTimeDown4_Cval_PT"
  pt_ShiftTimeUp1_Cval_PT/1 -> Inputs/159  "pt_ShiftTimeUp1_Cval_PT"
  pt_ShiftTimeUp2_Cval_PT/1 -> Inputs/160  "pt_ShiftTimeUp2_Cval_PT"
  pt_ShiftTimeUp3_Cval_PT/1 -> Inputs/161  "pt_ShiftTimeUp3_Cval_PT"
  pt_ShiftTimeUp4_Cval_PT/1 -> Inputs/162  "pt_ShiftTimeUp4_Cval_PT"
  pt_SysID_CCM/1 -> Inputs/163  "pt_SysID_CCM"
  pt_SysID_MCM/1 -> Inputs/164  "pt_SysID_MCM"
  pt_SysID_RCM/1 -> Inputs/165  "pt_SysID_RCM"
  pt_SysID_TCM/1 -> Inputs/166  "pt_SysID_TCM"
  pt_ThermoRoll_Rq/1 -> Inputs/167  "pt_ThermoRoll_Rq"
  pt_TopTrq_Rq_IPPC/1 -> Inputs/168  "pt_TopTrq_Rq_IPPC"
  pt_TrqConvLkup_Stat_PT/1 -> Inputs/169  "pt_TrqConvLkup_Stat_PT"
  pt_TrqConv_Cval_PT/1 -> Inputs/170  "pt_TrqConv_Cval_PT"
  pt_TrqConv_Stat_PT/1 -> Inputs/171  "pt_TrqConv_Stat_PT"
  pt_TxActlGrRatio_Cval_PT/1 -> Inputs/172  "pt_TxActlGrRatio_Cval_PT"
  pt_UpSpd_Cval_IPPC/1 -> Inputs/173  "pt_UpSpd_Cval_IPPC"
  pt_UseCase_Rq_IPPC/1 -> Inputs/174  "pt_UseCase_Rq_IPPC"
  pt_XBR_Rq_IPPC/1 -> Inputs/175  "pt_XBR_Rq_IPPC"
  drv_ign/1 -> Inputs/176  "drv_ign"
  Inputs/1 -> CPC5_SFUN_wrapper/1
  Outputs/1 -> ch_AccelPdlLoIdleSw_Stat/1  "<out_ch_AccelPdlLoIdleSw_Stat>"
  Outputs/2 -> ch_AccelPdlPosn_Cval/1  "<out_ch_AccelPdlPosn_Cval>"
  Outputs/3 -> ch_ActOffCond_Stat/1  "<out_ch_ActOffCond_Stat>"
  Outputs/4 -> ch_ActlEmotTrq_Cval/1  "<out_ch_ActlEmotTrq_Cval>"
  Outputs/5 -> ch_ActlEngPctTrq_Cval/1  "<out_ch_ActlEngPctTrq_Cval>"
  Outputs/6 -> ch_ActlMaxAvlRetPctTrq_Cval_CPC3/1  "<out_ch_ActlMaxAvlRetPctTrq_Cval_CPC3>"
  Outputs/7 -> ch_ActlRetPctTrq_Cval_CPC3/1  "<out_ch_ActlRetPctTrq_Cval_CPC3>"
  Outputs/8 -> ch_AutoSetSpdMd_Stat/1  "<out_ch_AutoSetSpdMd_Stat>"
  Outputs/9 -> ch_CC_Actv_Stat/1  "<out_ch_CC_Actv_Stat>"
  Outputs/10 -> ch_CC_Actvn_Stat/1  "<out_ch_CC_Actvn_Stat>"
  Outputs/11 -> ch_CC_BrkSpd_Cval/1  "<out_ch_CC_BrkSpd_Cval>"
  Outputs/12 -> ch_CC_FuncMode_Stat/1  "<out_ch_CC_FuncMode_Stat>"
  Outputs/13 -> ch_CC_HiResSetSpd_Cval/1  "<out_ch_CC_HiResSetSpd_Cval>"
  Outputs/14 -> ch_CC_HystSpd_Cval/1  "<out_ch_CC_HystSpd_Cval>"
  Outputs/15 -> ch_CC_SetSpd_Cval/1  "<out_ch_CC_SetSpd_Cval>"
  Outputs/16 -> ch_Clutch_Stat_CPC/1  "<out_ch_Clutch_Stat_CPC>"
  Outputs/17 -> ch_DeclSens_Cval_PT/1  "<out_ch_DeclSens_Cval_PT>"
  Outputs/18 -> ch_DispAutoMan_Rq_CPC/1  "<out_ch_DispAutoMan_Rq_CPC>"
  Outputs/19 -> ch_DispEngSp_Rq/1  "<out_ch_DispEngSp_Rq>"
  Outputs/20 -> ch_DispEngStSp_Stat/1  "<out_ch_DispEngStSp_Stat>"
  Outputs/21 -> ch_DrvDirec2_Stat_CPC/1  "<out_ch_DrvDirec2_Stat_CPC>"
  Outputs/22 -> ch_DrvDirec_Stat_TCM_PT/1  "<out_ch_DrvDirec_Stat_TCM_PT>"
  Outputs/23 -> ch_EngPctTrqDrv_Rq/1  "<out_ch_EngPctTrqDrv_Rq>"
  Outputs/24 -> ch_EngRPM_Cval_CPC3/1  "<out_ch_EngRPM_Cval_CPC3>"
  Outputs/25 -> ch_EngRefTrq_Cval/1  "<out_ch_EngRefTrq_Cval>"
  Outputs/26 -> ch_EngShutDownMSS_Stat/1  "<out_ch_EngShutDownMSS_Stat>"
  Outputs/27 -> ch_EngStSp_Stat/1  "<out_ch_EngStSp_Stat>"
  Outputs/28 -> ch_ExtAccel_Rq_CPC/1  "<out_ch_ExtAccel_Rq_CPC>"
  Outputs/29 -> ch_ExtBrkStat_Rq_CPC/1  "<out_ch_ExtBrkStat_Rq_CPC>"
  Outputs/30 -> ch_FanSpdPct_Cval_PT/1  "<out_ch_FanSpdPct_Cval_PT>"
  Outputs/31 -> ch_FanSpd_Cval_PT/1  "<out_ch_FanSpd_Cval_PT>"
  Outputs/32 -> ch_FuncLmpRET_Rq/1  "<out_ch_FuncLmpRET_Rq>"
  Outputs/33 -> ch_GrShift_Stat_PT/1  "<out_ch_GrShift_Stat_PT>"
  Outputs/34 -> ch_HB_Rq_Stat_CPC/1  "<out_ch_HB_Rq_Stat_CPC>"
  Outputs/35 -> ch_LastGrRlsRsn_Stat/1  "<out_ch_LastGrRlsRsn_Stat>"
  Outputs/36 -> ch_MC_E3_Cval_CPC/1  "<out_ch_MC_E3_Cval_CPC>"
  Outputs/37 -> ch_NomFrictEngPctTrq_Cval/1  "<out_ch_NomFrictEngPctTrq_Cval>"
  Outputs/38 -> ch_PtRt_Cval_CH/1  "<out_ch_PtRt_Cval_CH>"
  Outputs/39 -> ch_RetPctTrqActl2_Cval_CPC3/1  "<out_ch_RetPctTrqActl2_Cval_CPC3>"
  Outputs/40 -> ch_RetRefTrq_Cval/1  "<out_ch_RetRefTrq_Cval>"
  Outputs/41 -> ch_RetSwPos_Rq_STSR/1  "<out_ch_RetSwPos_Rq_STSR>"
  Outputs/42 -> ch_RetTrqMd_Stat_CPC3/1  "<out_ch_RetTrqMd_Stat_CPC3>"
  Outputs/43 -> ch_RetTrq_Cval_PT/1  "<out_ch_RetTrq_Cval_PT>"
  Outputs/44 -> ch_SLDrvMdSw_Stat/1  "<out_ch_SLDrvMdSw_Stat>"
  Outputs/45 -> ch_ShiftPrg_Stat/1  "<out_ch_ShiftPrg_Stat>"
  Outputs/46 -> ch_SrvBrkSw_Stat/1  "<out_ch_SrvBrkSw_Stat>"
  Outputs/47 -> ch_TargetEngTrqCpc_Rq/1  "<out_ch_TargetEngTrqCpc_Rq>"
  Outputs/48 -> ch_TrqConvLkup_Stat_PT/1  "<out_ch_TrqConvLkup_Stat_PT>"
  Outputs/49 -> ch_TrqConv_Cval_PT/1  "<out_ch_TrqConv_Cval_PT>"
  Outputs/50 -> ch_TrqConv_Stat_PT/1  "<out_ch_TrqConv_Stat_PT>"
  Outputs/51 -> ch_TxActlGrRatio_Cval/1  "<out_ch_TxActlGrRatio_Cval>"
  Outputs/52 -> ch_TxClutchPctSlp_Cval_CPC/1  "<out_ch_TxClutchPctSlp_Cval_CPC>"
  Outputs/53 -> ch_TxCurrGr_Stat/1  "<out_ch_TxCurrGr_Stat>"
  Outputs/54 -> ch_TxDrvlineEngg_Stat_CPC/1  "<out_ch_TxDrvlineEngg_Stat_CPC>"
  Outputs/55 -> ch_TxInShaftSpd_Cval_CPC/1  "<out_ch_TxInShaftSpd_Cval_CPC>"
  Outputs/56 -> ch_TxOutShaftSpd_Cval_CPC/1  "<out_ch_TxOutShaftSpd_Cval_CPC>"
  Outputs/57 -> ch_TxShftIP_Stat_CPC/1  "<out_ch_TxShftIP_Stat_CPC>"
  Outputs/58 -> ch_VehSpd_Cval_CPC/1  "<out_ch_VehSpd_Cval_CPC>"
  Outputs/59 -> pt_ACC_CtrlDmnt_Stat/1  "<out_pt_ACC_CtrlDmnt_Stat>"
  Outputs/60 -> pt_ATC_Ctrl_Stat_PT/1  "<out_pt_ATC_Ctrl_Stat_PT>"
  Outputs/61 -> pt_AccelPdlKickDnSw_Rq/1  "<out_pt_AccelPdlKickDnSw_Rq>"
  Outputs/62 -> pt_AccelPdlLoIdleSw_Stat/1  "<out_pt_AccelPdlLoIdleSw_Stat>"
  Outputs/63 -> pt_AccelPdlPosn_Cval/1  "<out_pt_AccelPdlPosn_Cval>"
  Outputs/64 -> pt_AmbTemp_Cval_PT/1  "<out_pt_AmbTemp_Cval_PT>"
  Outputs/65 -> pt_AutoSetSpdMd_Stat/1  "<out_pt_AutoSetSpdMd_Stat>"
  Outputs/66 -> pt_BS_Brk_Cval/1  "<out_pt_BS_Brk_Cval>"
  Outputs/67 -> pt_BrkPdlPosn3_Cval/1  "<out_pt_BrkPdlPosn3_Cval>"
  Outputs/68 -> pt_CC_Actvn_Stat_PT/1  "<out_pt_CC_Actvn_Stat_PT>"
  Outputs/69 -> pt_CC_FuncMode_Stat/1  "<out_pt_CC_FuncMode_Stat>"
  Outputs/70 -> pt_CC_HystSpd2_Cval/1  "<out_pt_CC_HystSpd2_Cval>"
  Outputs/71 -> pt_CC_HystSpd_Cval/1  "<out_pt_CC_HystSpd_Cval>"
  Outputs/72 -> pt_CC_LoHystSpd2_Cval/1  "<out_pt_CC_LoHystSpd2_Cval>"
  Outputs/73 -> pt_CC_LoHystSpd_Cval/1  "<out_pt_CC_LoHystSpd_Cval>"
  Outputs/74 -> pt_CC_Md_Stat/1  "<out_pt_CC_Md_Stat>"
  Outputs/75 -> pt_CC_SaveSetSpd_Rs/1  "<out_pt_CC_SaveSetSpd_Rs>"
  Outputs/76 -> pt_CC_SetSpd3_Cval/1  "<out_pt_CC_SetSpd3_Cval>"
  Outputs/77 -> pt_CC_SetSpd_Cval/1  "<out_pt_CC_SetSpd_Cval>"
  Outputs/78 -> pt_CC_SetSpd_Estm_Cval/1  "<out_pt_CC_SetSpd_Estm_Cval>"
  Outputs/79 -> pt_CPC_IdleCond_Stat_PT/1  "<out_pt_CPC_IdleCond_Stat_PT>"
  Outputs/80 -> pt_ClutchCls_Stat_PT/1  "<out_pt_ClutchCls_Stat_PT>"
  Outputs/81 -> pt_ClutchOpn_Rq_CPC/1  "<out_pt_ClutchOpn_Rq_CPC>"
  Outputs/82 -> pt_ClutchOpn_Stat_PT/1  "<out_pt_ClutchOpn_Stat_PT>"
  Outputs/83 -> pt_CoolLvl_Stat_PT/1  "<out_pt_CoolLvl_Stat_PT>"
  Outputs/84 -> pt_CstValIPPC_Stat/1  "<out_pt_CstValIPPC_Stat>"
  Outputs/85 -> pt_CurrManGr_Stat_PT/1  "<out_pt_CurrManGr_Stat_PT>"
  Outputs/86 -> pt_CurvSpd_Stat/1  "<out_pt_CurvSpd_Stat>"
  Outputs/87 -> pt_CutoffFreqSurgDamp_Cval_PT/1  "<out_pt_CutoffFreqSurgDamp_Cval_PT>"
  Outputs/88 -> pt_DPF_InhbtRegen_Rq_PT/1  "<out_pt_DPF_InhbtRegen_Rq_PT>"
  Outputs/89 -> pt_DateTmDay_Cval_ICUC/1  "<out_pt_DateTmDay_Cval_ICUC>"
  Outputs/90 -> pt_DateTmHour_Cval_ICUC/1  "<out_pt_DateTmHour_Cval_ICUC>"
  Outputs/91 -> pt_DateTmMinute_Cval_ICUC/1  "<out_pt_DateTmMinute_Cval_ICUC>"
  Outputs/92 -> pt_DateTmMonth_Cval_ICUC/1  "<out_pt_DateTmMonth_Cval_ICUC>"
  Outputs/93 -> pt_DateTmSecond_Cval_ICUC/1  "<out_pt_DateTmSecond_Cval_ICUC>"
  Outputs/94 -> pt_DateTmYear_Cval_ICUC/1  "<out_pt_DateTmYear_Cval_ICUC>"
  Outputs/95 -> pt_DipHystSpd_Cval/1  "<out_pt_DipHystSpd_Cval>"
  Outputs/96 -> pt_DisturbanceTrq_Cal/1  "<out_pt_DisturbanceTrq_Cal>"
  Outputs/97 -> pt_DrvFriction_Cval_PT/1  "<out_pt_DrvFriction_Cval_PT>"
  Outputs/98 -> pt_DynWhlRadius_Cval/1  "<out_pt_DynWhlRadius_Cval>"
  Outputs/99 -> pt_EcoRollMd_Stat/1  "<out_pt_EcoRollMd_Stat>"
  Outputs/100 -> pt_EcoRollNeu_Rq_PT/1  "<out_pt_EcoRollNeu_Rq_PT>"
  Outputs/101 -> pt_EngBrk1_Rq_PT/1  "<out_pt_EngBrk1_Rq_PT>"
  Outputs/102 -> pt_EngBrk2_Rq_PT/1  "<out_pt_EngBrk2_Rq_PT>"
  Outputs/103 -> pt_EngCrk_Stat/1  "<out_pt_EngCrk_Stat>"
  Outputs/104 -> pt_EngExtStart_Stat_PT/1  "<out_pt_EngExtStart_Stat_PT>"
  Outputs/105 -> pt_EngIdle_Stat_PT/1  "<out_pt_EngIdle_Stat_PT>"
  Outputs/106 -> pt_EngIgn_Stat_PT/1  "<out_pt_EngIgn_Stat_PT>"
  Outputs/107 -> pt_EngSpd_Rq_PT/1  "<out_pt_EngSpd_Rq_PT>"
  Outputs/108 -> pt_EngStrtr_Stat_PT/1  "<out_pt_EngStrtr_Stat_PT>"
  Outputs/109 -> pt_EngTrq_Rq_PT/1  "<out_pt_EngTrq_Rq_PT>"
  Outputs/110 -> pt_EngZeroTrq_Stat_PT/1  "<out_pt_EngZeroTrq_Stat_PT>"
  Outputs/111 -> pt_Fan_Rq_PT/1  "<out_pt_Fan_Rq_PT>"
  Outputs/112 -> pt_FuelLvl_Cval/1  "<out_pt_FuelLvl_Cval>"
  Outputs/113 -> pt_FuelMapSel_Rq_PT/1  "<out_pt_FuelMapSel_Rq_PT>"
  Outputs/114 -> pt_GaimSurgDamp_Cval_PT/1  "<out_pt_GaimSurgDamp_Cval_PT>"
  Outputs/115 -> pt_GovType_Stat_PT/1  "<out_pt_GovType_Stat_PT>"
  Outputs/116 -> pt_HiResAccelPdlPosn_Cval/1  "<out_pt_HiResAccelPdlPosn_Cval>"
  Outputs/117 -> pt_IPPC_Md2_Stat/1  "<out_pt_IPPC_Md2_Stat>"
  Outputs/118 -> pt_IPPC_Md_Rq/1  "<out_pt_IPPC_Md_Rq>"
  Outputs/119 -> pt_IgnSw_Stat_SCA/1  "<out_pt_IgnSw_Stat_SCA>"
  Outputs/120 -> pt_IntrUrbMd_Stat/1  "<out_pt_IntrUrbMd_Stat>"
  Outputs/121 -> pt_KickDn_Stat_PT/1  "<out_pt_KickDn_Stat_PT>"
  Outputs/122 -> pt_LimGovDroopSpd_Cval/1  "<out_pt_LimGovDroopSpd_Cval>"
  Outputs/123 -> pt_LocalMinuteOffset_Cval_ICUC/1  "<out_pt_LocalMinuteOffset_Cval_ICUC>"
  Outputs/124 -> pt_MaxEngSpd_Cval_PT/1  "<out_pt_MaxEngSpd_Cval_PT>"
  Outputs/125 -> pt_MinEngSpd_Cval_PT/1  "<out_pt_MinEngSpd_Cval_PT>"
  Outputs/126 -> pt_MomntOver_Rq_PT/1  "<out_pt_MomntOver_Rq_PT>"
  Outputs/127 -> pt_NeuRangeGroup_Rq_PT/1  "<out_pt_NeuRangeGroup_Rq_PT>"
  Outputs/128 -> pt_NeuSplitGroup_Rq_PT/1  "<out_pt_NeuSplitGroup_Rq_PT>"
  Outputs/129 -> pt_NeuSw_Stat_PT/1  "<out_pt_NeuSw_Stat_PT>"
  Outputs/130 -> pt_ObsDrvFriction_Cval_PT/1  "<out_pt_ObsDrvFriction_Cval_PT>"
  Outputs/131 -> pt_ObsSel_Cval/1  "<out_pt_ObsSel_Cval>"
  Outputs/132 -> pt_PTO_EstmTrq_Cval/1  "<out_pt_PTO_EstmTrq_Cval>"
  Outputs/133 -> pt_PrkBrk_Stat_PT/1  "<out_pt_PrkBrk_Stat_PT>"
  Outputs/134 -> pt_RegenActv_Rq_CPC/1  "<out_pt_RegenActv_Rq_CPC>"
  Outputs/135 -> pt_RetSwPosn2_Stat_PT/1  "<out_pt_RetSwPosn2_Stat_PT>"
  Outputs/136 -> pt_RetTrq_Rq_PT/1  "<out_pt_RetTrq_Rq_PT>"
  Outputs/137 -> pt_RlsSelGr_Rq_PT/1  "<out_pt_RlsSelGr_Rq_PT>"
  Outputs/138 -> pt_RoadGrad_Cval_PT/1  "<out_pt_RoadGrad_Cval_PT>"
  Outputs/139 -> pt_RoadGrad_Stat_PT/1  "<out_pt_RoadGrad_Stat_PT>"
  Outputs/140 -> pt_SPEEDO_ZeSig_Stat_PT/1  "<out_pt_SPEEDO_ZeSig_Stat_PT>"
  Outputs/141 -> pt_SelGr_Rq_PT/1  "<out_pt_SelGr_Rq_PT>"
  Outputs/142 -> pt_ShiftMd_Stat/1  "<out_pt_ShiftMd_Stat>"
  Outputs/143 -> pt_ShiftPrg_Stat/1  "<out_pt_ShiftPrg_Stat>"
  Outputs/144 -> pt_ShiftSprtEng_Rq_PT/1  "<out_pt_ShiftSprtEng_Rq_PT>"
  Outputs/145 -> pt_SpdFtAxleLtWhl_Cval/1  "<out_pt_SpdFtAxleLtWhl_Cval>"
  Outputs/146 -> pt_SpdFtAxleRtWhl_Cval/1  "<out_pt_SpdFtAxleRtWhl_Cval>"
  Outputs/147 -> pt_SpdR_AxleLtWhl_Cval/1  "<out_pt_SpdR_AxleLtWhl_Cval>"
  Outputs/148 -> pt_SpdR_AxleRtWhl_Cval/1  "<out_pt_SpdR_AxleRtWhl_Cval>"
  Outputs/149 -> pt_SrvBrkSw_Stat_PT/1  "<out_pt_SrvBrkSw_Stat_PT>"
  Outputs/150 -> pt_SurgeDamp_Stat_PT/1  "<out_pt_SurgeDamp_Stat_PT>"
  Outputs/151 -> pt_SysID_CPC3/1  "<out_pt_SysID_CPC3>"
  Outputs/152 -> pt_TargetEngTrqETP_Rq_PT/1  "<out_pt_TargetEngTrqETP_Rq_PT>"
  Outputs/153 -> pt_TargetEngTrqRQV_Rq_PT/1  "<out_pt_TargetEngTrqRQV_Rq_PT>"
  Outputs/154 -> pt_TargetEngTrq_Rq_PT/1  "<out_pt_TargetEngTrq_Rq_PT>"
  Outputs/155 -> pt_ThermoHt_Rq_PT/1  "<out_pt_ThermoHt_Rq_PT>"
  Outputs/156 -> pt_ThermoMgt_Stat_PT/1  "<out_pt_ThermoMgt_Stat_PT>"
  Outputs/157 -> pt_TotalVehDist_Cval_DIAG/1  "<out_pt_TotalVehDist_Cval_DIAG>"
  Outputs/158 -> pt_TrlrDet_Stat/1  "<out_pt_TrlrDet_Stat>"
  Outputs/159 -> pt_TrqLim_Cval_CPC/1  "<out_pt_TrqLim_Cval_CPC>"
  Outputs/160 -> pt_VehMtn_Stat_PT/1  "<out_pt_VehMtn_Stat_PT>"
  Outputs/161 -> pt_VehSpd_Cval_CPC/1  "<out_pt_VehSpd_Cval_CPC>"
  Outputs/162 -> pt_VehSpd_Cval_PT/1  "<out_pt_VehSpd_Cval_PT>"
  Outputs/163 -> pt_VehWeight_Cval_PT/1  "<out_pt_VehWeight_Cval_PT>"
  Outputs/164 -> pt_VehWeight_Stat_PT/1  "<out_pt_VehWeight_Stat_PT>"
  Outputs/165 -> pt_WtrPmp_Rq_PT/1  "<out_pt_WtrPmp_Rq_PT>"
  Outputs/166 -> pt_XBR_Stat_PT/1  "<out_pt_XBR_Stat_PT>"
  Outputs/167 -> pt_XSS_Stat/1  "<out_pt_XSS_Stat>"
  Outputs/168 -> cpc_Ignition/1  "<out_cpc_Ignition>"
  Outputs/169 -> cpc_TrqDecIdx/1  "<out_cpc_TrqDecIdx>"
  Outputs/170 -> cpc_ag_g_EngTargetSpeed/1  "<out_cpc_ag_g_EngTargetSpeed>"
  Outputs/171 -> cpc_ag_m_FiltTrqRatio/1  "<out_cpc_ag_m_FiltTrqRatio>"
  Outputs/172 -> cpc_cc_p_CcSecure_LowSwitchOnVehSpd_u8/1  "<out_cpc_cc_p_CcSecure_LowSwitchOnVehSpd_u8>"
  CPC5_SFUN_wrapper/1 -> Outputs/1
